simulink model "FOC_IM"  (R2021a)
settings: Solver=VariableStepAuto  StartTime=0.0  StopTime=10.0  RelTol=1e-3
undefined symbols (not defined in the file or in its folder): csat, DiscIntNeverNeededParam, fc, h, Ki, Kp, Lm, Lr, p, Rr, Tvect
libraries: spsCurrentMeasurementLib x3, spsVoltageMeasurementLib x3, spsDCVoltageSourceLib x1, fl_lib x1, spsAsynchronousMachinepuUnitsLib x1, spsUniversalBridgeLib x1
settings Model: Creator=ACER  LastModifiedBy=ACER

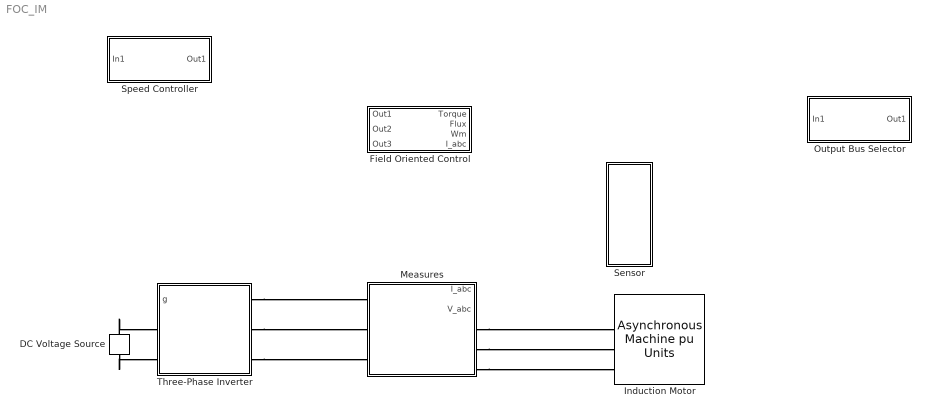
== system FOC_IM ==
  DC Voltage Source : spsDCVoltageSourceLib/DC Voltage Source  Amplitude=100  Measurements=None
  Field Oriented Control : Subsystem
  Induction Motor : spsAsynchronousMachinepuUnitsLib/Asynchronous Machine pu Units  RotorType=Squirrel-cage  PresetModel=No  MechanicalLoad=Torque Tm  ShowDetailedParameters=on  ReferenceFrame=Rotor  Units=pu  MeasurementBus=off  NominalParameters=[3730 460 60]  VoltageRatio=1  Stator=[0.01965 0.0397]  Rotor=[0.01909 0.0397]  Cage1=[0.01909 0.0397]  Cage2=[0.01909 0.0397]  Lm=1.354  Mechanical=[0.09526 0.05479 2]  PolePairs=2  InitialConditions="[ 1,0   0,0,0   0,0,0 ]"  SimulateSaturation=off  Saturation="[0.212,0.4201,0.8125,1.0979,1.4799,2.2457,3.2586,4.5763,6.4763 ;   0.5,0.7,0.9,1,1.1,1.2 ,1.3,1.4,1.5]"  LoadFlowParameters=0  TsPowergui=0  TsBlock=-1  IterativeModel=Trapezoidal non iterative  IterativeDiscreteModel=Trapezoidal non iterative  Pmec=0
      settings: SourceProductBaseCode=PS
  "Measures " : Subsystem
  Output Bus Selector : Subsystem
  Sensor : Subsystem
  Speed Controller : Subsystem
  Three-Phase Inverter : Subsystem
  connections:
  "Measures "/RConn3 -- Induction Motor/LConn3
  "Measures "/RConn2 -- Induction Motor/LConn2
  "Measures "/RConn1 -- Induction Motor/LConn1
  Three-Phase Inverter/RConn1 -- "Measures "/LConn1
  Three-Phase Inverter/RConn2 -- "Measures "/LConn2
  Three-Phase Inverter/RConn3 -- "Measures "/LConn3
  DC Voltage Source/RConn1 -- Three-Phase Inverter/LConn1
  DC Voltage Source/LConn1 -- Three-Phase Inverter/LConn2

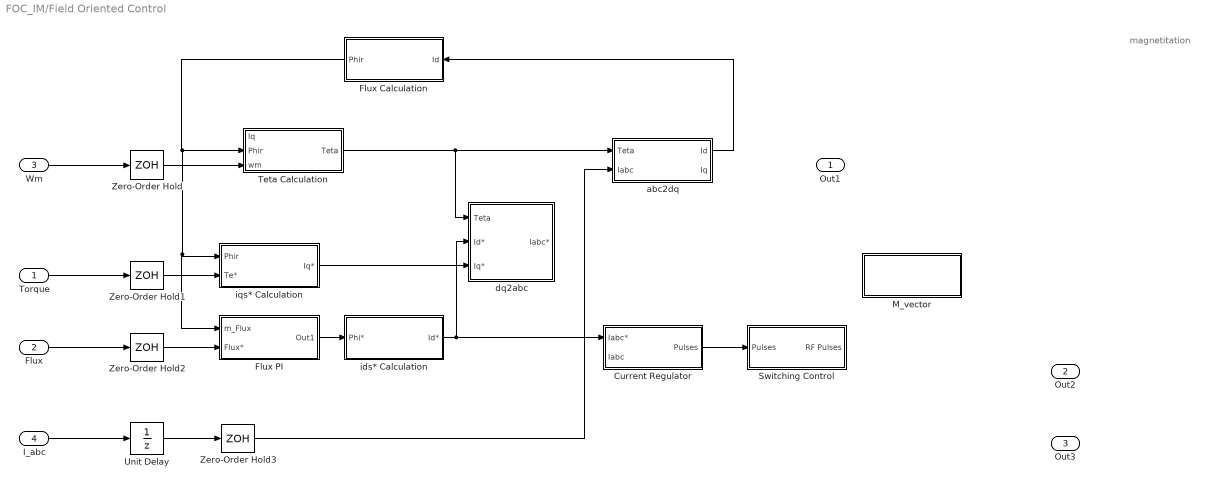
== system FOC_IM/Field Oriented Control ==
  note: magnetitation
  Torque : Inport
  Flux : Inport  Port=2
  Wm : Inport  Port=3
  I_abc : Inport  Port=4
  Current Regulator : Subsystem
  Flux Calculation : Subsystem
  Flux PI : Subsystem
  M_vector : Subsystem
  "Switching Control " : Subsystem
  Teta Calculation : Subsystem
  Unit Delay : UnitDelay  SampleTime=-1  HasFrameUpgradeWarning=on
  Zero-Order Hold{,1..3} (4 alike) : ZeroOrderHold  SampleTime=Tvect
  abc2dq : Subsystem
  dq2abc : Subsystem
  ids* Calculation : Subsystem
  iqs* Calculation : Subsystem
  Out1 : Outport
  Out2 : Outport  Port=2
  Out3 : Outport  Port=3
  wires:
  iqs* Calculation/1(Iq*) -> dq2abc/3(Iq*)
  Wm/1 -> Zero-Order Hold/1
  Torque/1 -> Zero-Order Hold1/1
  Flux/1 -> Zero-Order Hold2/1
  I_abc/1 -> Unit Delay/1
  Zero-Order Hold1/1 -> iqs* Calculation/2(Te*)
  Zero-Order Hold2/1 -> Flux PI/2(Flux*)
  Flux PI/1(Out1) -> ids* Calculation/1(Phi*)
  ids* Calculation/1(Id*) -> dq2abc/2(Id*), Current Regulator/1(Iabc*)
  Zero-Order Hold/1 -> Teta Calculation/3(wm)
  Teta Calculation/1(Teta) -> dq2abc/1(Teta), abc2dq/1(Teta)
  abc2dq/1(Id) -> Flux Calculation/1(Id)
  Flux Calculation/1(Phir) -> Flux PI/1(m_Flux), iqs* Calculation/1(Phir), Teta Calculation/2(Phir)
  Unit Delay/1 -> Zero-Order Hold3/1
  Zero-Order Hold3/1 -> abc2dq/2(Iabc)
  Current Regulator/1(Pulses) -> "Switching Control "/1(Pulses)

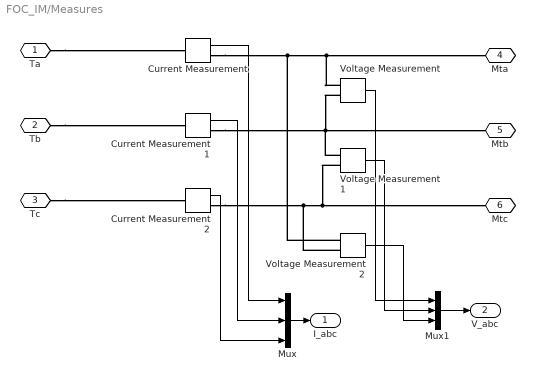
== system FOC_IM/Measures  ==
  Current Measurement : spsCurrentMeasurementLib/Current Measurement  PhasorSimulation=off  OutputType=Complex  PSBequivalent=0
  Current Measurement1 : spsCurrentMeasurementLib/Current Measurement  PhasorSimulation=off  OutputType=Complex  PSBequivalent=0
  Current Measurement2 : spsCurrentMeasurementLib/Current Measurement  PhasorSimulation=off  OutputType=Complex  PSBequivalent=0
  Mux : Mux  Inputs=3
  Mux1 : Mux  Inputs=3
  Voltage Measurement : spsVoltageMeasurementLib/Voltage Measurement  PhasorSimulation=off  OutputType=Complex  PSBequivalent=0
  Voltage Measurement1 : spsVoltageMeasurementLib/Voltage Measurement  PhasorSimulation=off  OutputType=Complex  PSBequivalent=0
  Voltage Measurement2 : spsVoltageMeasurementLib/Voltage Measurement  PhasorSimulation=off  OutputType=Complex  PSBequivalent=0
  Ta : PMIOPort  Side=Left
  Tb : PMIOPort  Port=2  Side=Left
  Tc : PMIOPort  Port=3  Side=Left
  "Mta " : PMIOPort  Port=4  Side=Right
  Mtb : PMIOPort  Port=5  Side=Right
  Mtc : PMIOPort  Port=6  Side=Right
  I_abc : Outport
  V_abc : Outport  Port=2
  wires:
  Current Measurement/1 -> Mux/1
  Current Measurement1/1 -> Mux/2
  Current Measurement2/1 -> Mux/3
  Mux/1 -> I_abc/1
  Voltage Measurement/1 -> Mux1/1
  Voltage Measurement1/1 -> Mux1/2
  Voltage Measurement2/1 -> Mux1/3
  Mux1/1 -> V_abc/1
  connections:
  Ta/RConn1 -- Current Measurement/LConn1
  Current Measurement/RConn1 -- Voltage Measurement2/LConn1 -- Voltage Measurement/LConn1 -- "Mta "/RConn1
  Tb/RConn1 -- Current Measurement1/LConn1
  Current Measurement1/RConn1 -- Voltage Measurement1/LConn1 -- Voltage Measurement/LConn2 -- Mtb/RConn1
  Tc/RConn1 -- Current Measurement2/LConn1
  Current Measurement2/RConn1 -- Voltage Measurement2/LConn2 -- Voltage Measurement1/LConn2 -- Mtc/RConn1

== system FOC_IM/Output Bus Selector ==
  In1 : Inport
  Out1 : Outport
  wires:
  In1/1 -> Out1/1

== system FOC_IM/Sensor ==

== system FOC_IM/Speed Controller ==
  In1 : Inport
  Out1 : Outport
  wires:
  In1/1 -> Out1/1

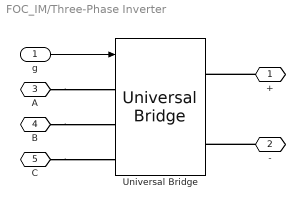
== system FOC_IM/Three-Phase Inverter ==
  g : Inport
  Universal Bridge : spsUniversalBridgeLib/Universal Bridge  Arms=3  SnubberResistance=1e5  SnubberCapacitance=inf  Device=IGBT / Diodes  Ron=1e-3  Lon=0  ForwardVoltages="[  0  0  ]"  ForwardVoltage=0  GTOparameters=[ 10e-6 , 20e-6 ]  IGBTparameters=[ 1e-6 , 2e-6 ]  Measurements=None  Measurements_2=None  converterType=Rectifier
  + : PMIOPort  Side=Left
  - : PMIOPort  Port=2  Side=Left
  A : PMIOPort  Port=3  Side=Right
  B : PMIOPort  Port=4  Side=Right
  C : PMIOPort  Port=5  Side=Right
  wires:
  g/1 -> Universal Bridge/1
  connections:
  +/RConn1 -- Universal Bridge/RConn1
  -/RConn1 -- Universal Bridge/RConn2
  A/RConn1 -- Universal Bridge/LConn1
  B/RConn1 -- Universal Bridge/LConn2
  C/RConn1 -- Universal Bridge/LConn3

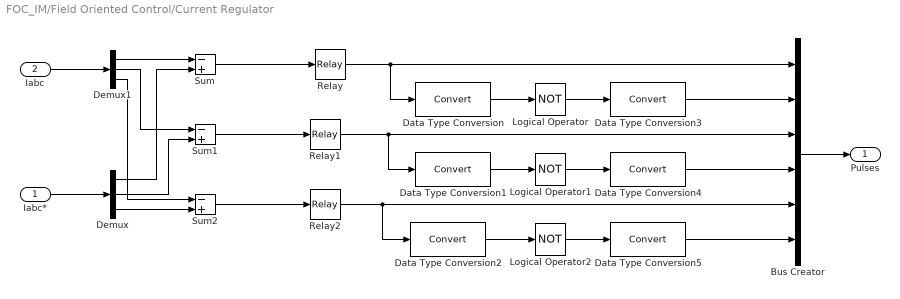
== system FOC_IM/Field Oriented Control/Current Regulator ==
  Iabc* : Inport
  Iabc : Inport  Port=2
  Bus Creator : BusCreator  Inputs=6
  Data Type Conversion{,1..5} (6 alike) : DataTypeConversion
  Demux : Demux  Outputs=3
      settings: DisplayOption=none
  Demux1 : Demux  Outputs=3
      settings: DisplayOption=none
  Logical Operator : Logic  Operator=NOT  AllPortsSameDT=off  OutDataTypeStr=boolean
  Logical Operator1 : Logic  Operator=NOT  AllPortsSameDT=off  OutDataTypeStr=boolean
  Logical Operator2 : Logic  Operator=NOT  AllPortsSameDT=off  OutDataTypeStr=boolean
  Relay : Relay  OnSwitchValue=h/2  OffSwitchValue=-h/2
  Relay1 : Relay  OnSwitchValue=h/2  OffSwitchValue=-h/2
  Relay2 : Relay  OnSwitchValue=h/2  OffSwitchValue=-h/2
  Sum : Sum  Inputs=-+
  Sum1 : Sum  Inputs=-+
  Sum2 : Sum  Inputs=-+
  Pulses : Outport
  wires:
  Iabc*/1 -> Demux/1
  Iabc/1 -> Demux1/1
  Demux1/1 -> Sum/1
  Demux1/2 -> Sum1/1
  Demux1/3 -> Sum2/1
  Demux/1 -> Sum/2
  Demux/2 -> Sum1/2
  Demux/3 -> Sum2/2
  Sum/1 -> Relay/1
  Sum1/1 -> Relay1/1
  Sum2/1 -> Relay2/1
  Data Type Conversion/1 -> Logical Operator/1
  Logical Operator/1 -> Data Type Conversion3/1
  Logical Operator1/1 -> Data Type Conversion4/1
  Data Type Conversion1/1 -> Logical Operator1/1
  Logical Operator2/1 -> Data Type Conversion5/1
  Data Type Conversion2/1 -> Logical Operator2/1
  Relay/1 -> Data Type Conversion/1, Bus Creator/1
  Data Type Conversion3/1 -> Bus Creator/2
  Relay1/1 -> Data Type Conversion1/1, Bus Creator/3
  Data Type Conversion4/1 -> Bus Creator/4
  Relay2/1 -> Data Type Conversion2/1, Bus Creator/5
  Data Type Conversion5/1 -> Bus Creator/6
  Bus Creator/1 -> Pulses/1

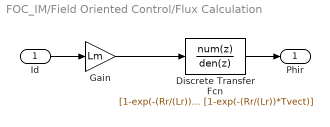
== system FOC_IM/Field Oriented Control/Flux Calculation ==
  Id : Inport
  Discrete Transfer Fcn : DiscreteTransferFcn  Numerator=[1-exp(-(Rr/(Lr))*Tvect)]  Denominator=[1-exp(-(Rr/(Lr))*Tvect)]  SampleTime=Tvect
  Gain : Gain  Gain=Lm
  Phir : Outport
  wires:
  Id/1 -> Gain/1
  Gain/1 -> Discrete Transfer Fcn/1
  Discrete Transfer Fcn/1 -> Phir/1

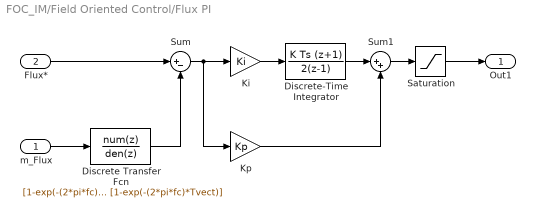
== system FOC_IM/Field Oriented Control/Flux PI ==
  m_Flux : Inport
  Flux* : Inport  Port=2
  Discrete Transfer Fcn : DiscreteTransferFcn  Numerator=[1-exp(-(2*pi*fc)*Tvect)]  Denominator=[1-exp(-(2*pi*fc)*Tvect)]  SampleTime=Tvect
  Discrete-Time Integrator : DiscreteIntegrator  IntegratorMethod=Integration: Trapezoidal  SampleTime=Tvect  LimitOutput=on  UpperSaturationLimit=csat(2)  LowerSaturationLimit=csat(1)  ICPrevOutput=DiscIntNeverNeededParam  ICPrevScaledInput=DiscIntNeverNeededParam
  Ki : Gain  Gain=Ki
  Kp : Gain  Gain=Kp
  Saturation : Saturate  UpperLimit=csat(2)  LowerLimit=cast(1)
  Sum : Sum  Inputs=|+-
  Sum1 : Sum  Inputs=|++
  Out1 : Outport
  wires:
  Flux*/1 -> Sum/1
  m_Flux/1 -> Discrete Transfer Fcn/1
  Discrete Transfer Fcn/1 -> Sum/2
  Sum/1 -> Kp/1, Ki/1
  Kp/1 -> Sum1/2
  Discrete-Time Integrator/1 -> Sum1/1
  Ki/1 -> Discrete-Time Integrator/1
  Sum1/1 -> Saturation/1
  Saturation/1 -> Out1/1

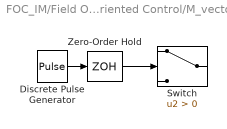
== system FOC_IM/Field Oriented Control/M_vector ==
  Discrete Pulse Generator : DiscretePulseGenerator  Period=8  PulseWidth=2  SampleTime=Tvect
  Switch : Switch  Criteria=u2 > Threshold
  Zero-Order Hold : ZeroOrderHold  SampleTime=Tvect
  wires:
  Discrete Pulse Generator/1 -> Zero-Order Hold/1
  Zero-Order Hold/1 -> Switch/2

== system FOC_IM/Field Oriented Control/Switching Control  ==
  Pulses : Inport
  Controlled Current Source : fl_lib/Electrical/Electrical Sources/Controlled Current Source
  RF Pulses : Outport
  wires:
  Pulses/1 -> RF Pulses/1

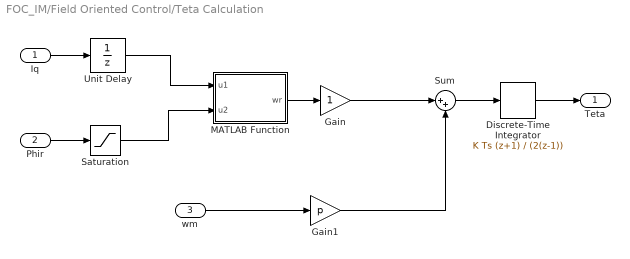
== system FOC_IM/Field Oriented Control/Teta Calculation ==
  Iq : Inport
  Phir : Inport  Port=2
  wm : Inport  Port=3
  Discrete-Time Integrator : DiscreteIntegrator  IntegratorMethod=Integration: Trapezoidal  SampleTime=Tvect  ICPrevOutput=DiscIntNeverNeededParam  ICPrevScaledInput=DiscIntNeverNeededParam
  Gain : Gain
  Gain1 : Gain  Gain=p
  MATLAB Function : MATLAB Function  TreatAsAtomicUnit=on
  Saturation : Saturate  UpperLimit=inf  LowerLimit=1e-3
  Sum : Sum  Inputs=|++
  Unit Delay : UnitDelay  SampleTime=-1  HasFrameUpgradeWarning=on
  Teta : Outport
  wires:
  Iq/1 -> Unit Delay/1
  Phir/1 -> Saturation/1
  Unit Delay/1 -> MATLAB Function/1(u1)
  Saturation/1 -> MATLAB Function/2(u2)
  MATLAB Function/1(wr) -> Gain/1
  wm/1 -> Gain1/1
  Gain/1 -> Sum/1
  Gain1/1 -> Sum/2
  Sum/1 -> Discrete-Time Integrator/1
  Discrete-Time Integrator/1 -> Teta/1

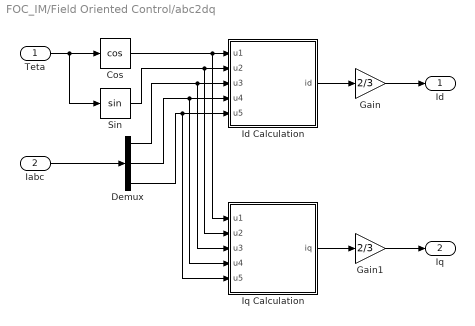
== system FOC_IM/Field Oriented Control/abc2dq ==
  Teta : Inport
  Iabc : Inport  Port=2
  Cos : Trigonometry  Operator=cos
  Demux : Demux  Outputs=3
      settings: DisplayOption=none
  Gain : Gain  Gain=2/3
  Gain1 : Gain  Gain=2/3
  Id Calculation : MATLAB Function  TreatAsAtomicUnit=on
  Iq Calculation : MATLAB Function  TreatAsAtomicUnit=on
  Sin : Trigonometry
  Id : Outport
  Iq : Outport  Port=2
  wires:
  Teta/1 -> Sin/1, Cos/1
  Iabc/1 -> Demux/1
  Cos/1 -> Iq Calculation/1(u1), Id Calculation/1(u1)
  Sin/1 -> Iq Calculation/2(u2), Id Calculation/2(u2)
  Demux/1 -> Iq Calculation/3(u3), Id Calculation/3(u3)
  Demux/2 -> Iq Calculation/4(u4), Id Calculation/4(u4)
  Demux/3 -> Iq Calculation/5(u5), Id Calculation/5(u5)
  Id Calculation/1(id) -> Gain/1
  Iq Calculation/1(iq) -> Gain1/1
  Gain/1 -> Id/1
  Gain1/1 -> Iq/1

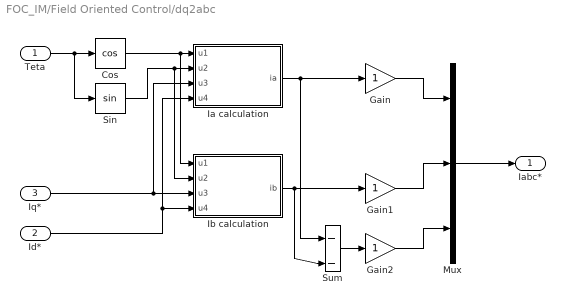
== system FOC_IM/Field Oriented Control/dq2abc ==
  Teta : Inport
  Id* : Inport  Port=2
  Iq* : Inport  Port=3
  Cos : Trigonometry  Operator=cos
  Gain : Gain
  Gain1 : Gain
  Gain2 : Gain
  Ia calculation : MATLAB Function  TreatAsAtomicUnit=on
  Ib calculation : MATLAB Function  TreatAsAtomicUnit=on
  Mux : Mux  Inputs=3
  Sin : Trigonometry
  Sum : Sum  Inputs=--
  Iabc* : Outport
  wires:
  Teta/1 -> Sin/1, Cos/1
  Cos/1 -> Ib calculation/1(u1), Ia calculation/1(u1)
  Sin/1 -> Ib calculation/2(u2), Ia calculation/2(u2)
  Iq*/1 -> Ib calculation/3(u3), Ia calculation/3(u3)
  Id*/1 -> Ib calculation/4(u4), Ia calculation/4(u4)
  Ia calculation/1(ia) -> Sum/1, Gain/1
  Ib calculation/1(ib) -> Sum/2, Gain1/1
  Sum/1 -> Gain2/1
  Gain2/1 -> Mux/3
  Gain1/1 -> Mux/2
  Gain/1 -> Mux/1
  Mux/1 -> Iabc*/1

== system FOC_IM/Field Oriented Control/ids* Calculation ==
  Phi* : Inport
  Gain : Gain  Gain=1/Lm
  Id* : Outport
  wires:
  Phi*/1 -> Gain/1
  Gain/1 -> Id*/1

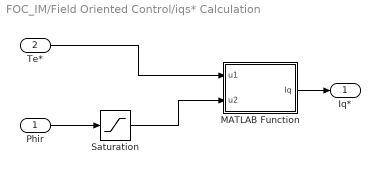
== system FOC_IM/Field Oriented Control/iqs* Calculation ==
  Phir : Inport
  Te* : Inport  Port=2
  MATLAB Function : MATLAB Function  TreatAsAtomicUnit=on
  Saturation : Saturate  UpperLimit=inf  LowerLimit=1e-3
  Iq* : Outport
  wires:
  Phir/1 -> Saturation/1
  Saturation/1 -> MATLAB Function/2(u2)
  Te*/1 -> MATLAB Function/1(u1)
  MATLAB Function/1(Iq) -> Iq*/1

== matlab function FOC_IM/Field Oriented Control/dq2abc/Ia calculation ==
  data: u1 input; ia output; u2 input; u3 input; u4 input
function ia = fcn(u1, u2, u3, u4)

ia = -u3*u2+u4*u1;

== matlab function FOC_IM/Field Oriented Control/iqs* Calculation/MATLAB Function ==
  data: u1 input; Iq output; u2 input
function Iq = fcn(u1, u2)

Iq* = (2/3)*(1/p)*(Lr/Lm)*u1/(u2+1e-3*0);

== matlab function FOC_IM/Field Oriented Control/dq2abc/Ib calculation ==
  data: u1 input; ib output; u2 input; u3 input; u4 input
function ib = fcn(u1, u2, u3, u4)

ib = (-u1+1.7320508*u2)*u4*0.5+(u2+1.7320508*u1)*u3*0.5;

== matlab function FOC_IM/Field Oriented Control/Teta Calculation/MATLAB Function ==
  data: u1 input; wr output; u2 input
function wr = fcn(u1, u2)

wr = Lm*u1/(u2*(Lr/Rr)+1e-3*0);

== matlab function FOC_IM/Field Oriented Control/abc2dq/Id Calculation ==
  data: u1 input; id output; u2 input; u3 input; u4 input; u5 input
function id = fcn(u1, u2, u3, u4, u5)

id = u1*u3+(1.73*u2-u1)*u4*0.5+(u1-1.73*u2)*u5*0.5;

== matlab function FOC_IM/Field Oriented Control/abc2dq/Iq Calculation ==
  data: u1 input; iq output; u2 input; u3 input; u4 input; u5 input
function iq = fcn(u1, u2, u3, u4, u5)

iq = -u2*u3+(u2+1.73*u1)*u4*0.5+(u2-1.73*u1)*u5*0.5;
